simulink library "Yaw_Ideal_Motor_Lib"  (Simulink 7.9)
settings: Solver=ode45  StartTime=0.0  StopTime=10.0  RelTol=1e-3
undefined symbols (not defined in the file): deg, gcbh, mech_rtmsupport, mech_support, s, WT_Params
libraries: mblibv1 x6, fl_lib x5, nesl_utility x3, Yaw_Gearbox_Lib x1
Description:
  | Copyright 2011 MathWorks, Inc.
settings Model: Creator=smiller  LastModifiedBy=smiller

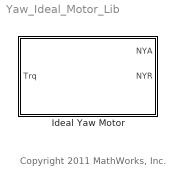
== system Yaw_Ideal_Motor_Lib ==
  note: Copyright 2011 MathWorks, Inc.
  Ideal Yaw Motor : Subsystem
      mask Display: image(imread('Yaw_Ideal_Motor_Horizontal_IMAGE.jpg'));

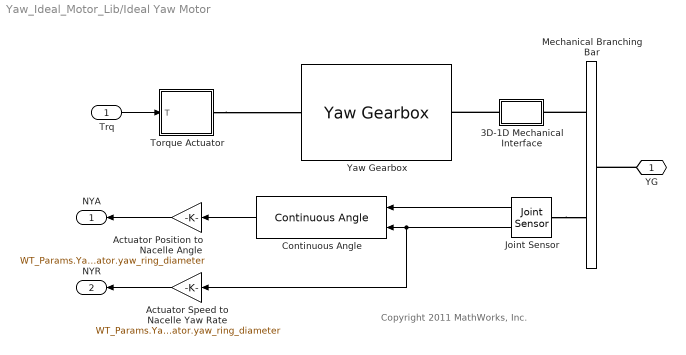
== system Yaw_Ideal_Motor_Lib/Ideal Yaw Motor ==
  note: Copyright 2011 MathWorks, Inc.
  Trq : Inport
  3D-1D Mechanical Interface : Subsystem
  Actuator Position to Nacelle Angle : Gain  Gain=WT_Params.Yaw_Actuator.yaw_gear_diameter/WT_Params.Yaw_Actuator.yaw_ring_diameter
  Actuator Speed to Nacelle Yaw Rate : Gain  Gain=WT_Params.Yaw_Actuator.yaw_gear_diameter/WT_Params.Yaw_Actuator.yaw_ring_diameter
  Continuous Angle : mblibv1/Utilities/Continuous Angle  rad=deg  rads=deg/s
  Joint Sensor : mblibv1/Sensors &  Actuators/Joint Sensor  UpdateFromCAD=off  PhysicalDomain=Mechanical  PortType=blob  Muxed=off  Pose=off  Angle=on  AngleUnits=deg  ArcVelocity=on  ArcVelocityUnits=deg/s  ArcAcceleration=off  ArcAccelerationUnits=deg/s^2  CoordPosition=on  CoordPositionUnits=m  Velocity=off  VelocityUnits=m/s  Acceleration=off  AccelerationUnits=m/s^2  Quaternion=on  QuaternionDT=off  QuaternionDDT=off  QuaternionUnits=off  OutputVector=[1]  ActiveIO=off  Width=2  DialogClass=MechanicalSensorBlock  Primitive=R1  Force=off  ForceUnits=N  Torque=off  TorqueUnits=N*m  ReferenceFrame=Absolute (World)  ReactionSensedSide=Base  ReactionReferenceFrame=Local (Body CS)  ReactionForce=off  ReactionForceUnits=N  ReactionMoment=off  ReactionMomentUnits=N*m
  Mechanical Branching Bar : mblibv1/Utilities/Mechanical Branching Bar  LConnTagsString=_newl0  RConnTagsString=SA0|SA1  UpdateFromCAD=off  DialogClass=MechanicalBranchingBarBlock  NumSAPorts=2
  Torque Actuator : Subsystem
      mask Display:
      | plot(400-[198.657636314574;187.5372000791;176.524559560751;165.725772507838;155.244837142898;145.182690602959;135.636236859729;126.697413481378;118.452306223496;110.980319976212;104.353414051689;98.6354091766174;93.8813728637222;90.1370890815176;87.4386173296598;85.811945366254;85.272738931537;85.8261908782356;87.4669711615554;90.1792781704262;93.9369909056548;98.7039205394262;104.434158933498;111.072520759669;118.555074964656;126.809760461083;135.75708011515;145.310866347487;155.379110974044;165.864851295207;176.667103899592;187.681837189509;192.988368326926],[283.691199740558;283.13774779386;281.49696751054;278.784660501669;275.026947766441;270.260018132669;264.529779738597;257.891417912426;250.40886370744;242.154178211013;233.206858556945;223.653072324609;213.584827698051;203.099087376889;192.296834772503;181.282101482586;170.160965409986;159.040529174513;148.027888656163;137.22910160325;126.748166238311;116.686019698372;107.139565955142;98.2007425767901;89.9556353189084;82.4836490716241;75.8567431471018;70.1387382720299;65.3847019591348;61.6404181769301;58.9419464250722;57.3152744616664;56.9214337615639])
      | plot(400-[85.209725657478;1.11807254143059;1.11807254143059], [170.435198815539;170.435198815539;171.380048850551])
      | plot(400-[283.691223012283;397.073227213696], [170.309218810871;170.309218810871])
      | plot(400-[153.301918180659;255.34572196193], [170.309218810871;170.309218810871])
      | plot(400-[198.654719861224;113.618216710165;198.654719861224], [85.2727156598121;170.309218810871;255.34572196193])
      | plot(400-[198.654719861224;153.301918180659;198.654719861224], [215.662020491436;170.309218810871;124.956417130306])
      | plot(400-[198.654719861224;283.691223012283;283.691223012283;187.316519441083;192.985619651154], [283.691223012283;283.691223012283;56.927214609459;56.927214609459;56.927214609459])
      | 
      | patch(400-[395.419739652425;395.419739652425;5.6843418860808e-14;0;395.419739652425;394.947314634919;0.472425017505884;0.472425017505941;394.947314634919;394.947314634919;395.419739652425], [340.618437621742;5.6843418860808e-14;0;340.618437621742;340.618437621742;340.146012604237;340.146012604237;0.472425017505884;0.472425017505884;340.146012604237;340.618437621742], [1;1;1])
      | ;
      | color('red');
      | port_label('RConn', 1,'R')
      | port_label('Input', 1,'T')
  Yaw Gearbox : Yaw_Gearbox_Lib/Yaw Gearbox  SystemSampleTime=-1
  YG : PMIOPort  Port=1  Side=Right
  NYA : Outport
  NYR : Outport  Port=2
  wires:
  Trq/1 -> Torque Actuator/1(T)
  Joint Sensor/2 -> Actuator Speed to Nacelle Yaw Rate/1, Continuous Angle/2
  Joint Sensor/1 -> Continuous Angle/1
  Continuous Angle/1 -> Actuator Position to Nacelle Angle/1
  Actuator Position to Nacelle Angle/1 -> NYA/1
  Actuator Speed to Nacelle Yaw Rate/1 -> NYR/1
  connections:
  3D-1D Mechanical Interface/LConn1 -- Yaw Gearbox/RConn1
  Torque Actuator/RConn1 -- Yaw Gearbox/LConn1
  Mechanical Branching Bar/RConn1 -- 3D-1D Mechanical Interface/RConn1
  Joint Sensor/LConn1 -- Mechanical Branching Bar/RConn2
  YG/RConn1 -- Mechanical Branching Bar/LConn1

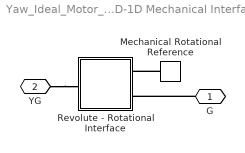
== system Yaw_Ideal_Motor_Lib/Ideal Yaw Motor/3D-1D Mechanical Interface ==
  Mechanical Rotational Reference : fl_lib/Mechanical/Rotational Elements/Mechanical Rotational Reference  t_Log=off  LocalVarNames=|t  LocalVarDescs=|t  LocalVarLogging=0
  Revolute - Rotational Interface : Subsystem  DialogController=MECH.DynMechDlgSource  LoadFcn=mech_rtmsupport('LoadFcn',gcbh);mech_support('LoadFcn',gcbh);  StartFcn=mech_support('StartFcn',gcbh);  StopFcn=mech_support('StopFcn',gcbh);  mask(Revolute - Rotational Interface){UpdateFromCAD=off, PMImportedID=, ClassName=RevoluteRotationalInterface, DialogClass=RevoluteRotationalInterface, Primitive=R1}
      mask prompts: UpdateFromCAD "UPDATE_FROM_CAD"; PMImportedID "PMIMPORTED_ID"; Primitive "Connected to primitive :"
      mask help:
      | Connects a revolute primitive in the Joint attached at port R to any two mechanical rotational nodes in a Simscape network. Exchanges rotational kinetic energy between a machine and a network without loss. The base (B) and follower (F) ports correspond to the same ports on the Joint. Connect to Joint block to see Connected to primitive list.
      |
      | To ensure model validity, do not place inertia elements in interfaced Simscape circuit.
      mask init:
      | mech_preinitmask ();
      | mech_support('MaskInit',gcbh)
      settings: CopyFcn=mech_rtmsupport('CopyFcn',gcbh);mech_support('CopyFcn',gcbh);  DeleteFcn=mech_rtmsupport('DeleteFcn',gcbh);mech_support('DeleteFcn',gcbh);  UndoDeleteFcn=mech_support('UndoDeleteFcn',gcbh);  ModelCloseFcn=mech_rtmsupport('ModelCloseFcn',gcbh);mech_support('ModelCloseFcn',gcbh);  PreSaveFcn=mech_rtmsupport('PreSaveFcn',gcbh);  PostSaveFcn=mech_rtmsupport('PostSaveFcn',gcbh);  NameChangeFcn=mech_support('NameChangeFcn',gcbh);  PreCopyFcn=mech_rtmsupport('PreCopyFcn',gcbh);  CloseFcn=mech_support('CloseFcn',gcbh);  PreDeleteFcn=mech_rtmsupport('PreDeleteFcn',gcbh);
      mask Help: web(mech_help('revoluterotationalinterface'))
      mask Display: image(mech_getIcon('revolute_interface.bmp', 'Mechanical'),'center','on');color('magenta');port_label('lconn',1,'B');port_label('lconn',2,'F');color('black');port_label('rconn',1,'R');
  G : PMIOPort  Port=1  Side=Left
  YG : PMIOPort  Port=2  Side=Right
  connections:
  YG/RConn1 -- Revolute - Rotational Interface/RConn1
  Mechanical Rotational Reference/LConn1 -- Revolute - Rotational Interface/LConn1
  G/RConn1 -- Revolute - Rotational Interface/LConn2

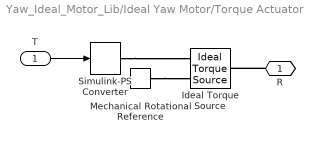
== system Yaw_Ideal_Motor_Lib/Ideal Yaw Motor/Torque Actuator ==
  T : Inport
  Ideal Torque Source : fl_lib/Mechanical/Mechanical Sources/Ideal Torque Source  w_Log=off  t_Log=off  LocalVarNames=|w|t  LocalVarDescs=|w|t  LocalVarLogging=[0 0]
  Mechanical Rotational Reference : fl_lib/Mechanical/Rotational Elements/Mechanical Rotational Reference  SystemSampleTime=-1  t_Log=off  LocalVarNames=|t  LocalVarDescs=|t  LocalVarLogging=0
  Simulink-PS Converter : nesl_utility/Simulink-PS Converter  SystemSampleTime=-1  PhysicalDomain=network_engine_domain  LeftPortType=input  RightPortType=output  SubClassName=ps_input  Unit=1  AffineConversion=off  InputFilterTimeConstant=.001  UdotUserProvided=0
  R : PMIOPort  Port=1  Side=Right
  wires:
  T/1 -> Simulink-PS Converter/1
  connections:
  Simulink-PS Converter/RConn1 -- Ideal Torque Source/RConn1
  Mechanical Rotational Reference/LConn1 -- Ideal Torque Source/RConn2
  R/RConn1 -- Ideal Torque Source/LConn1

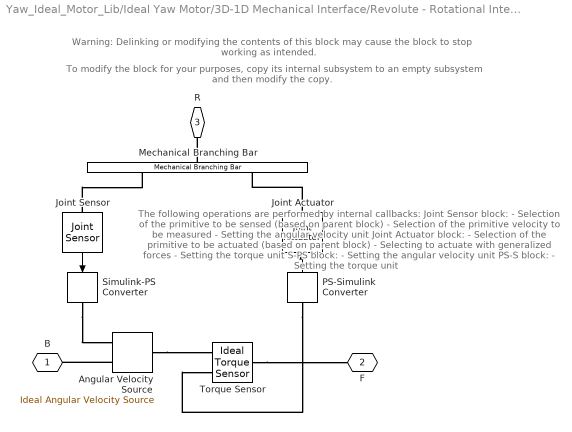
== system Yaw_Ideal_Motor_Lib/Ideal Yaw Motor/3D-1D Mechanical Interface/Revolute - Rotational Interface ==
  note: Warning: Delinking or modifying the contents of
      | this block may cause the block to stop working as intended.
  note: To modify the block for your purposes, copy its internal subsystem
      | to an empty subsystem and then modify the copy.
  note: The following operations are performed by internal callbacks:
      |
      | Joint Sensor block:
      |    - Selection of the primitive to be sensed (based on parent block)
      |    - Selection of the primitive velocity to be measured
      |    - Setting the angular velocity unit
      |
      | Joint Actuator block:
      |    - Selection of the primitive to be actuated (based on parent block)
      |    - Selecting to actuate with generalized forces
      |    - Setting the torque unit
      |
      | S-PS block:
      |    - Setting the angular velocity unit
      |
      | PS-S block:
      |    - Setting the torque unit
  Angular Velocity Source : fl_lib/Mechanical/Mechanical Sources/Ideal Angular Velocity Source  w_Log=off  t_Log=off  LocalVarNames=|torque|rel_velocity|power  LocalVarDescs=|Torque (N*m)|Relative velocity (rad/s)|Power generated by the sourcec(W)  LocalVarLogging=[0 0 0]
  Joint Actuator : mblibv1/Sensors &  Actuators/Joint Actuator  UpdateFromCAD=off  PhysicalDomain=Mechanical  PortType=blob  ActuationStyle=Force  AngleUnits=deg  ArcVelocityUnits=deg/s  ArcAccelerationUnits=deg/s^2  CoordPositionUnits=m  VelocityUnits=m/s  AccelerationUnits=m/s^2  ForceUnits=N  TorqueUnits=N*m  ActiveIO=off  Width=1  DialogClass=MechanicalActuatorBlock  Primitive=R1  ReferenceFrame=Absolute (World)
  Joint Sensor : mblibv1/Sensors &  Actuators/Joint Sensor  UpdateFromCAD=off  PhysicalDomain=Mechanical  PortType=blob  Muxed=on  Pose=off  Angle=off  AngleUnits=deg  ArcVelocity=on  ArcVelocityUnits=rad/s  ArcAcceleration=off  ArcAccelerationUnits=deg/s^2  CoordPosition=off  CoordPositionUnits=m  Velocity=off  VelocityUnits=m/s  Acceleration=off  AccelerationUnits=m/s^2  Quaternion=off  QuaternionDT=off  QuaternionDDT=off  QuaternionUnits=off  OutputVector=[1]  ActiveIO=off  Width=1  DialogClass=MechanicalSensorBlock  Primitive=R1  Force=off  ForceUnits=N  Torque=off  TorqueUnits=N*m  ReferenceFrame=Absolute (World)  ReactionSensedSide=Base  ReactionReferenceFrame=Absolute (World)  ReactionForce=off  ReactionForceUnits=N  ReactionMoment=off  ReactionMomentUnits=N*m
  Mechanical Branching Bar : mblibv1/Utilities/Mechanical Branching Bar  LConnTagsString=_newl0  RConnTagsString=SA0|SA1  UpdateFromCAD=off  DialogClass=MechanicalBranchingBarBlock  NumSAPorts=2
  PS-Simulink Converter : nesl_utility/PS-Simulink Converter  PhysicalDomain=network_engine_domain  LeftPortType=input  RightPortType=output  SubClassName=ps_output  Unit=N*m  AffineConversion=off
  Simulink-PS Converter : nesl_utility/Simulink-PS Converter  PhysicalDomain=network_engine_domain  LeftPortType=input  RightPortType=output  SubClassName=ps_input  Unit=rad/s  AffineConversion=off  InputFilterTimeConstant=.001  UdotUserProvided=1  SimscapeFilterOrder=1  InputFiltering=on
  Torque Sensor : fl_lib/Mechanical/Mechanical Sensors/Ideal Torque Sensor  w_Log=off  t_Log=off  LocalVarNames=|w|t  LocalVarDescs=|w|t  LocalVarLogging=[]
  B : PMIOPort  Port=1  Side=Left
  F : PMIOPort  Port=2  Side=Left
  R : PMIOPort  Port=3  Side=Right
  wires:
  PS-Simulink Converter/1 -> Joint Actuator/1
  Joint Sensor/1 -> Simulink-PS Converter/1
  connections:
  Joint Actuator/RConn1 -- Mechanical Branching Bar/RConn2
  Joint Sensor/LConn1 -- Mechanical Branching Bar/RConn1
  Mechanical Branching Bar/LConn1 -- R/RConn1
  Torque Sensor/LConn1 -- F/RConn1
  Simulink-PS Converter/RConn1 -- Angular Velocity Source/RConn1
  Angular Velocity Source/RConn2 -- B/RConn1
  Angular Velocity Source/LConn1 -- Torque Sensor/RConn1
  PS-Simulink Converter/LConn1 -- Torque Sensor/RConn2
